simulink model "UAVSim_v2018a"  (R2018a)
settings: Solver=VariableStepAuto  StartTime=0.0  StopTime=40  RelTol=1e-3
values from neighbouring files (symbols this model uses):
  A = [0 0 0 1 0 0 0 0 0 0 0 0 ... (first row only)    [UAV.m]
  B = [ 0 0 0 0 ... (first row only)    [UAV.m]
  Xref = [100 100 100 0 0 0 ]    [UAV.m]
undefined symbols (not defined in the file or in its folder): Kang, Keu, Kpv
settings Model: Creator=abiabdap  LastModifiedBy=abiabdap
settings DebuggingCC: LibraryContextMissingDiagnostic=warning
settings SFSimCC: SimUseLocalCustomCode=on
settings RTWCC: RTWUseLocalCustomCode=on

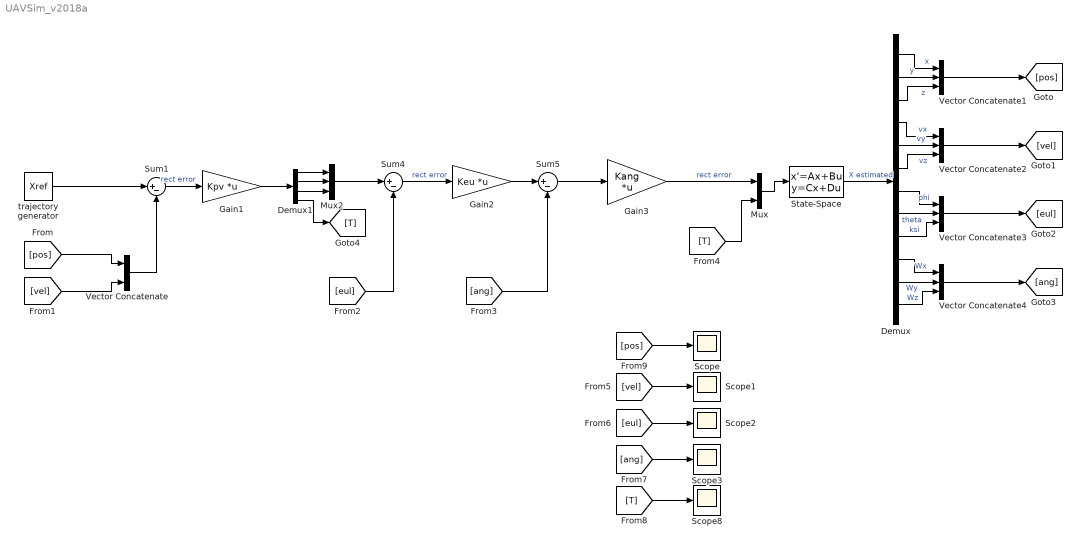
== system UAVSim_v2018a ==
  Demux : Demux  Outputs=12
  Demux1 : Demux
  Gain1 : Gain  Gain=Kpv  Multiplication=Matrix(K*u)
  Gain2 : Gain  Gain=Keu  Multiplication=Matrix(K*u)
  Gain3 : Gain  Gain=Kang  Multiplication=Matrix(K*u)
  Mux : Mux  Inputs=2
  Mux2 : Mux  Inputs=3
  Scope{,1..3,8} (5 alike) : Scope
  State-Space : StateSpace  A=A  B=B  C=eye(12)  D=zeros(12, 4)  InitialCondition=0
  Sum1 : Sum  Inputs=|+-
  Sum4 : Sum  Inputs=|+-
  Sum5 : Sum  Inputs=|+-
  Vector Concatenate : Concatenate
  Vector Concatenate{1..4} (4 alike) : Concatenate  NumInputs=3
  trajectory generator : Constant  Value=Xref
  wires:
  State-Space/1 -> Demux/1  "X estimated"
  trajectory generator/1 -> Sum1/1
  Sum1/1 -> Gain1/1  "rect error"
  [pos] -> Vector Concatenate/1
  [vel] -> Vector Concatenate/2
  Vector Concatenate/1 -> Sum1/2
  [eul] -> Sum4/2
  Sum4/1 -> Gain2/1  "rect error"
  Sum5/1 -> Gain3/1
  [ang] -> Sum5/2
  Gain2/1 -> Sum5/1
  Demux/1 -> Vector Concatenate1/1  "x"
  Demux/2 -> Vector Concatenate1/2  "y"
  Demux/3 -> Vector Concatenate1/3  "z"
  Vector Concatenate1/1 -> [pos]
  Demux/4 -> Vector Concatenate2/1  "vx"
  Demux/5 -> Vector Concatenate2/2  "vy"
  Demux/6 -> Vector Concatenate2/3  "vz"
  Demux/7 -> Vector Concatenate3/1  "phi"
  Demux/8 -> Vector Concatenate3/2  "theta"
  Demux/9 -> Vector Concatenate3/3  "ksi"
  Demux/10 -> Vector Concatenate4/1  "Wx"
  Demux/11 -> Vector Concatenate4/2  "Wy"
  Demux/12 -> Vector Concatenate4/3  "Wz"
  Vector Concatenate4/1 -> [ang]
  Vector Concatenate3/1 -> [eul]
  Vector Concatenate2/1 -> [vel]
  Gain1/1 -> Demux1/1
  Mux/1 -> State-Space/1
  Gain3/1 -> Mux/1  "rect error"
  Demux1/1 -> Mux2/1
  Demux1/2 -> Mux2/2
  Demux1/3 -> Mux2/3
  Mux2/1 -> Sum4/1
  Demux1/4 -> [T]
  [T] -> Mux/2
  [pos] -> Scope/1
  [vel] -> Scope1/1
  [eul] -> Scope2/1
  [ang] -> Scope3/1
  [T] -> Scope8/1
